simulink model "sampleModel258"  (R2021b)
settings: Solver=VariableStepAuto  StartTime=0.0  StopTime=10.0  RelTol=1e-3
undefined symbols (not defined in the file or in its folder): Newton, Raphson
libraries: simulink x13, slpidlib x2
settings Model: Creator=user  LastModifiedBy=user

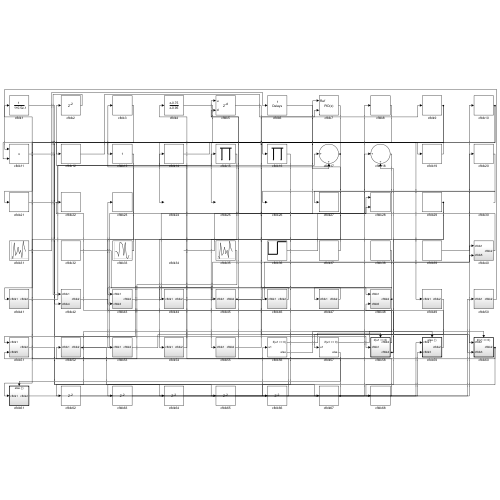
[thumbnail: Simulink's stored preview of the top-level diagram]
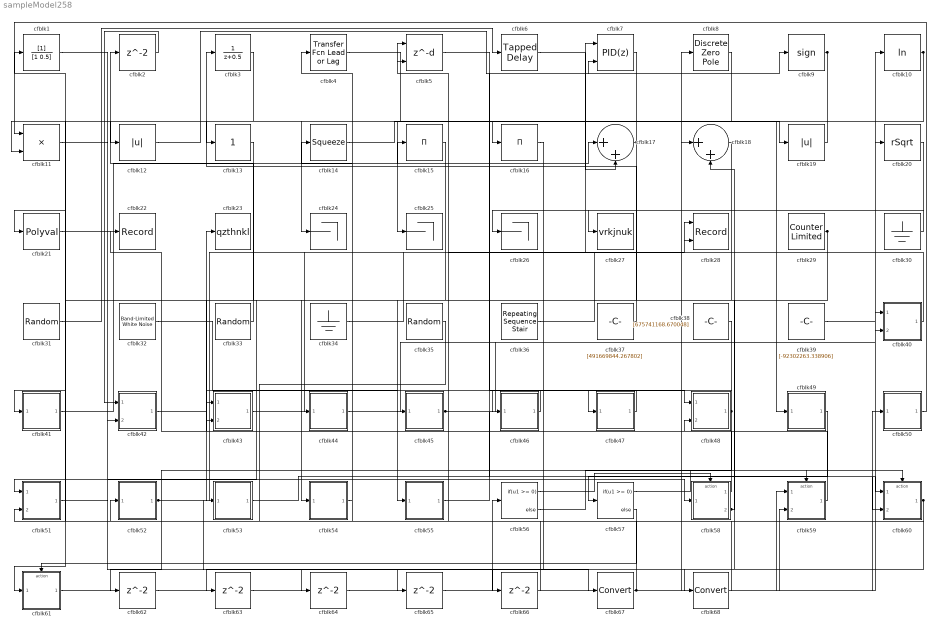
== system sampleModel258 ==
  cfblk1 : DiscreteFilter  SampleTime=1
  cfblk10 : Math  Operator=log  SaturateOnIntegerOverflow=on
  cfblk11 : Product  Inputs=**
  cfblk12 : Abs
  cfblk13 : simulink/Math Operations/Slider Gain  gain=1  low=0  high=2
  cfblk14 : Squeeze
  cfblk15 : Product  Inputs=*
  cfblk16 : Product  Inputs=*
  cfblk17 : Sum  Inputs=|++
  cfblk18 : Sum  Inputs=|++
  cfblk19 : Abs
  cfblk{2,62..66} (6 alike) : Delay  SampleTime=1
  cfblk20 : Sqrt  Operator=rSqrt  AlgorithmType=Newton-Raphson  SaturateOnIntegerOverflow=on
  cfblk21 : Polyval  Coefs=[ +2.081618890e-019, -1.441693666e-014, +4.719686976e-010, -8.536869453e-006, +1.621573104e-001, -8.087801117e+001 ]
  cfblk22 : Record  FileSettingsInternal="{\"entries\":[{\"content\":{\"excelSettings\":{\"content\":{},\"type\":\"Streamout.ExcelSettings\"}},\"type\":\"Streamout.FileSettingStorage\",\"uuid\":\"0ec8da23-2161-4a9d-a8a6-f1492471a594\"}],\"packageUris\":[\"http://schema.mathworks.com/mf0/streamout_blocks/R2020a\"],\"version\":\"1.0\"}"  SignalsInternal="{\"entries\":[{\"content\":{\"signals\":[{\"content\":{\"blockPath\":[\"sampleModel258/cfblk22\"],\"channel\":[],\"dimensions\":[1,1],\"domain\":\"sampleModel258/cfblk22\",\"lineColor\":\"#d95319\",\"plots\":[1],\"port\":1,\"sid\":[\"\"],\"signalID\":10667,\"signalName\":\"cfblk59\"},\"type\":\"RecordBlkView.Signal\",\"uuid\":\"13791875-5c6d-4bb0-95fb-77da70401f61\"}]},\"type\":\"RecordBlkView.InputSignals\",\"uuid\":\"91cc19b9-e580-4e4a-b56f-bdf48a70d35d\"}],\"packageUris\":[\"http://schema.mathworks.com/mf0/streamout_blocks/R2020a\"],\"version\":\"1.0\"}"  VisualizationBindings="{\"sparklinesplugin\":{\"info\":[{\"bindingParametersList\":[],\"subplotID\":1}]}}"
  cfblk23 : ToWorkspace  VariableName=qzthnkl  SaveFormat=Timeseries  SampleTime=-1
  cfblk24 : Terminator
  cfblk25 : Terminator
  cfblk26 : Terminator
  cfblk27 : ToWorkspace  VariableName=vrkjnuk  SaveFormat=Timeseries  SampleTime=-1
  cfblk28 : Record  FileSettingsInternal="{\"entries\":[{\"content\":{\"excelSettings\":{\"content\":{},\"type\":\"Streamout.ExcelSettings\"}},\"type\":\"Streamout.FileSettingStorage\",\"uuid\":\"56d646ea-4447-4100-bd41-ac8c1b7b2ac5\"}],\"packageUris\":[\"http://schema.mathworks.com/mf0/streamout_blocks/R2020a\"],\"version\":\"1.0\"}"  Layout=[1 1]  SignalsInternal="{\"entries\":[{\"content\":{\"signals\":[{\"content\":{\"blockPath\":[\"sampleModel258/cfblk28\"],\"channel\":[],\"dimensions\":[1],\"domain\":\"sampleModel258/cfblk28\",\"lineColor\":\"#a2142f\",\"plots\":[1],\"port\":1,\"sid\":[\"\"],\"signalID\":10671,\"signalName\":\"cfblk36\"},\"type\":\"RecordBlkView.Signal\",\"uuid\":\"d70a7a42-212c-47d6-9b85-39228d5a4333\"},{\"content\":{\"blockPath\":[\"sampleModel258/cfblk28\"],\"channel\":[],\"dimensions\":[1],\"domain\":\"sampleModel258/cfblk28\",\"lineColor\":\"#139fff\",\"plots\":[1],\"port\":2,\"sid\":[\"\"],\"signalID\":10675,\"signalName\":\"cfblk43\"},\"type\":\"RecordBlkView.Signal\",\"uuid\":\"f3014852-2a86-4845-a5c4-efbef73839ba\"}]},\"type\":\"RecordBlkView.InputSignals\",\"uuid\":\"fac5a7e7-c933-4a0b-812e-c4fec9d164f8\"}],\"packageUris\":[\"http://schema.mathworks.com/mf0/streamout_blocks/R2020a\"],\"version\":\"1.0\"}"  VisualizationBindings="{\"xyplotplugin\":{\"info\":[{\"series\":[{\"bindingParametersList\":[{\"parameter\":\"X-Axis\",\"signalID\":10671,\"signalName\":\"cfblk36\"},{\"parameter\":\"Y-Axis\",\"signalID\":10675,\"signalName\":\"cfblk43\"}],\"seriesID\":24969}],\"subplotID\":1}]}}"  CompatibilityTag=XY
  cfblk29 : simulink/Sources/Counter Limited  uplimit=[963.000000]  tsamp=-1
  cfblk3 : DiscreteTransferFcn  SampleTime=1
  cfblk30 : Ground
  cfblk31 : UniformRandomNumber  Minimum=[-523047582.222967]  Maximum=[2283029263.965306]  Seed=[18053115.000000]  SampleTime=0.1
  cfblk32 : simulink/Sources/Band-Limited White Noise  Cov=[465247779.470941]  Ts=0.1  seed=[5161787319.000000]
  cfblk33 : RandomNumber  Mean=[-77347.122146]  Variance=[42546.750938]  Seed=[226363169.000000]  SampleTime=0.1
  cfblk34 : Ground
  cfblk35 : UniformRandomNumber  Minimum=[-1875152426.312598]  Maximum=[3895215180.124573]  Seed=[16865050.000000]  SampleTime=0.1
  cfblk36 : simulink/Sources/Repeating Sequence Stair  OutValues=[-492891194.523507, -158957976.510578]  tsamp=-1  OutMin=[]  OutMax=[]  OutDataTypeStr=double  OutputDataTypeScalingMode=double  OutDataType=fixdt(0,8)  ConRadixGroup=Best Precision: Vector-wise  OutScaling=2^-12
  cfblk37 : Constant  Value=[491669844.267802]  SampleTime=1
  cfblk38 : Constant  Value=[675741168.670048]  SampleTime=1
  cfblk39 : Constant  Value=[-92302263.338906]  SampleTime=1
  cfblk4 : simulink/Discrete/Transfer Fcn Lead or Lag  PoleZ=0.95  ZeroZ=0.75  ICPrevOutput=0.0  ICPrevInput=0.0  DoSatur=off
      settings: SourceProductBaseCode=SL
  cfblk40 : Subsystem
  cfblk41 : Subsystem
  cfblk42 : Subsystem
  cfblk43 : Subsystem
  cfblk44 : Subsystem
  cfblk45 : Subsystem
  cfblk46 : Subsystem
  cfblk47 : Subsystem
  cfblk48 : Subsystem
  cfblk49 : Subsystem
  cfblk5 : Delay  DelayLengthSource=Input port  SampleTime=1
      settings: InputPortMap=u0,p1
  cfblk50 : Subsystem
  cfblk51 : Subsystem
  cfblk52 : Subsystem
  cfblk53 : Subsystem
  cfblk54 : Subsystem
  cfblk55 : Subsystem
  cfblk56 : If  IfExpression=u1 >= 0  SampleTime=1
  cfblk57 : If  IfExpression=u1 >= 0  SampleTime=1
  cfblk58 : Subsystem  TreatAsAtomicUnit=on
  cfblk59 : Subsystem  TreatAsAtomicUnit=on
  cfblk6 : simulink/Discrete/Tapped Delay  vinit=0.0  samptime=-1  NumDelays=1  DelayOrder=Oldest  includeCurrent=off
  cfblk60 : Subsystem  TreatAsAtomicUnit=on
  cfblk61 : Subsystem  TreatAsAtomicUnit=on
  cfblk67 : DataTypeConversion
  cfblk68 : DataTypeConversion
  cfblk7 : slpidlib/PID Controller (2DOF)  Controller=PID  Form=Parallel  TimeDomain=Discrete-time  UseExternalTs=off  SampleTime=1  IntegratorMethod=Forward Euler  FilterMethod=Forward Euler  ControllerParametersSource=internal  P=1  I=1  D=0  UseFilter=on  N=100  b=1  c=1  TunerSelectOption=Transfer Function Based (PID Tuner App)  InitialConditionSource=internal  InitialConditionForIntegrator=0  InitialConditionForFilter=0  DifferentiatorICPrevScaledInput=0  ExternalReset=none  TrackingMode=off  Kt=1  LimitOutput=off  SatLimitsSource=internal  UpperSaturationLimit=inf  LowerSaturationLimit=-inf  LinearizeAsGain=off  AntiWindupMode=none  Kb=1  POutMin=[]  POutMax=[]  IOutMin=[]  IOutMax=[]  DOutMin=[]  DOutMax=[]  NOutMin=[]  NOutMax=[]  bOutMin=[]  bOutMax=[]  cOutMin=[]  cOutMax=[]  SumOutMin=[]  SumOutMax=[]  SaturationOutMin=[]  SaturationOutMax=[]  PParamMin=[]  PParamMax=[]  IParamMin=[]  IParamMax=[]  DParamMin=[]  DParamMax=[]  NParamMin=[]  NParamMax=[]  bParamMin=[]  bParamMax=[]  cParamMin=[]  cParamMax=[]  KbParamMin=[]  KbParamMax=[]  KtParamMin=[]  KtParamMax=[]  KbOutMin=[]  KbOutMax=[]  KtOutMin=[]  KtOutMax=[]  IntegratorOutMin=[]  IntegratorOutMax=[]  FilterOutMin=[]  FilterOutMax=[]  SumI1OutMin=[]  SumI1OutMax=[]  SumI2OutMin=[]  SumI2OutMax=[]  SumI3OutMin=[]  SumI3OutMax=[]  SumI4OutMin=[]  SumI4OutMax=[]  SumDOutMin=[]  SumDOutMax=[]  Sum1OutMin=[]  Sum1OutMax=[]  Sum2OutMin=[]  Sum2OutMax=[]  Sum3OutMin=[]  Sum3OutMax=[]  DifferentiatorOutMin=[]  DifferentiatorOutMax=[]  FilterDiffOutCoefMin=[]  FilterDiffOutCoefMax=[]  ReciprocalOutMin=[]  ReciprocalOutMax=[]  SumDenOutMin=[]  SumDenOutMax=[]  SumNumOutMin=[]  SumNumOutMax=[]  DivideOutMin=[]  DivideOutMax=[]  UdiffTsProdOutMin=[]  UdiffTsProdOutMax=[]  NTsProdOutMin=[]  NTsProdOutMax=[]  UintegralTsProdOutMin=[]  UintegralTsProdOutMax=[]  UngainTsProdOutMin=[]  UngainTsProdOutMax=[]  IntegratorContinuousStateAttributes=''  IntegratorStateMustResolveToSignalObject=off  IntegratorRTWStateStorageClass=Auto  FilterContinuousStateAttributes=''  FilterStateMustResolveToSignalObject=off  FilterRTWStateStorageClass=Auto  ParallelPVariant=InternalParameters  IdealPVariant=Disabled  IVariant=InternalParameters  DVariant=InternalParameters  bVariant=InternalParameters  cVariant=InternalParameters  IntegratorVariant=Discrete  SatVariant=Disabled  AWVariant=Passthrough  PCopyVariant=Disabled  TRVariant=Disabled  FdbkBlocksVariant=Forward  IdealPFdbkVariant=Disabled  SatFdbkVariant=Disabled  DerivativeFilterVariant=ForwardEulerFilter  NVariant=InternalParameters  NCopyVariant=Disabled  FilterICVariant=InternalICsFilter  IntegratorICVariant=InternalICs  ExternalResetVariant=Disabled  TRSumVariant=Passthrough  SumFdbkVariant=Disabled  SumVariant=Sum_PID  TsampFilterVariant=InternalTs  TsampNgainVariant=Passthrough  TsampIntegralVariant=Passthrough  ExternalSaturationOutDataTypeStr=Inherit: Same as second input
      settings: SourceProductBaseCode=SL
  cfblk8 : DiscreteZeroPole  Poles=[0 0.5]  Gain=1
  cfblk9 : Signum
  wires:
  cfblk30/1 -> cfblk27/1
  cfblk10/1 -> cfblk25/1, cfblk11/2
  cfblk33/1 -> cfblk2/1
  cfblk39/1 -> cfblk10/1
  cfblk15/1 -> cfblk51/1(cfblk1)
  cfblk38/1 -> cfblk54/1(cfblk1)
  cfblk41/1(cfblk2) -> cfblk15/1
  cfblk2/1 -> cfblk42/1(cfblk1)
  cfblk9/1 -> cfblk24/1, cfblk42/2(cfblk4)
  cfblk60/1(cfblk2) -> cfblk52/1(cfblk1), cfblk63/1
  cfblk31/1 -> cfblk6/1
  cfblk36/1 -> cfblk28/1
  cfblk20/1 -> cfblk26/1
  cfblk61/1(cfblk2) -> cfblk20/1
  cfblk37/1 -> cfblk3/1
  cfblk48/1(cfblk2) -> cfblk47/1(cfblk1), cfblk62/1
  cfblk12/1 -> cfblk9/1
  cfblk50/1(cfblk2) -> cfblk11/1
  cfblk19/1 -> cfblk16/1
  cfblk7/1 -> cfblk12/1
  cfblk35/1 -> cfblk51/2(cfblk5)
  cfblk21/1 -> cfblk17/1
  cfblk6/1 -> cfblk17/2
  cfblk40/1(cfblk2) -> cfblk5/1
  cfblk14/1 -> cfblk19/1
  cfblk58/1(cfblk2) -> cfblk23/1
  cfblk8/1 -> cfblk41/1(cfblk1)
  cfblk1/1 -> cfblk67/1
  cfblk54/1(cfblk2) -> cfblk4/1
  cfblk17/1 -> cfblk13/1, cfblk45/1(cfblk1)
  cfblk52/1(cfblk2) -> cfblk8/1, cfblk65/1
  cfblk13/1 -> cfblk61/1(cfblk1)
  cfblk11/1 -> cfblk58/1(cfblk1)
  cfblk18/1 -> cfblk53/1(cfblk1)
  cfblk5/1 -> cfblk48/1(cfblk1)
  cfblk45/1(cfblk2) -> cfblk40/1(cfblk1), cfblk60/2(cfblk3)
  cfblk46/1(cfblk2) -> cfblk43/1(cfblk1)
  cfblk58/2(cfblk4) -> cfblk48/2(cfblk5), cfblk18/2
  cfblk43/1(cfblk2) -> cfblk28/2
  cfblk32/1 -> cfblk55/1(cfblk1)
  cfblk29/1 -> cfblk44/1(cfblk1), cfblk68/1
  cfblk4/1 -> cfblk49/1(cfblk1)
  cfblk34/1 -> cfblk7/1
  cfblk53/1(cfblk2) -> cfblk60/1(cfblk1)
  cfblk42/1(cfblk2) -> cfblk43/2(cfblk3)
  cfblk55/1(cfblk2) -> cfblk7/2
  cfblk47/1(cfblk2) -> cfblk46/1(cfblk1)
  cfblk49/1(cfblk2) -> cfblk57/1
  cfblk44/1(cfblk2) -> cfblk40/2(cfblk5)
  cfblk3/1 -> cfblk21/1
  cfblk59/1(cfblk2) -> cfblk22/1
  cfblk56/1 -> cfblk58/Action
  cfblk56/2 -> cfblk59/Action
  cfblk57/1 -> cfblk60/Action
  cfblk57/2 -> cfblk61/Action
  cfblk62/1 -> cfblk59/1(cfblk1)
  cfblk63/1 -> cfblk56/1
  cfblk51/1(cfblk2) -> cfblk64/1
  cfblk64/1 -> cfblk59/2(cfblk3)
  cfblk65/1 -> cfblk18/1
  cfblk16/1 -> cfblk66/1
  cfblk66/1 -> cfblk14/1
  cfblk67/1 -> cfblk5/2, cfblk50/1(cfblk1)
  cfblk68/1 -> cfblk1/1

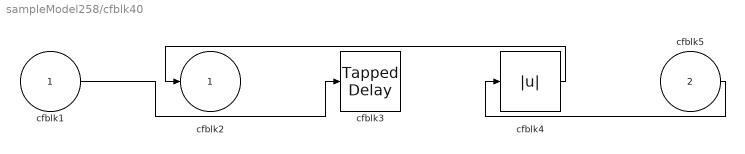
== system sampleModel258/cfblk40 ==
  cfblk1 : Inport
  cfblk5 : Inport  Port=2
  cfblk3 : simulink/Discrete/Tapped Delay  vinit=0.0  samptime=-1  NumDelays=1  DelayOrder=Oldest  includeCurrent=off
  cfblk4 : Abs
  cfblk2 : Outport
  wires:
  cfblk4/1 -> cfblk2/1
  cfblk1/1 -> cfblk3/1
  cfblk5/1 -> cfblk4/1

== system sampleModel258/cfblk41 ==
  cfblk1 : Inport
  cfblk3 : Abs
  cfblk2 : Outport
  wires:
  cfblk1/1 -> cfblk3/1
  cfblk3/1 -> cfblk2/1

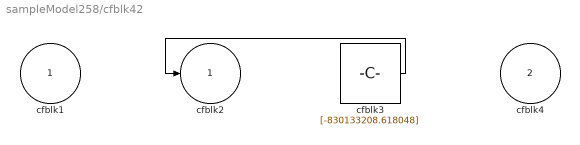
== system sampleModel258/cfblk42 ==
  cfblk1 : Inport
  cfblk4 : Inport  Port=2
  cfblk3 : Constant  Value=[-830133208.618048]  SampleTime=1
  cfblk2 : Outport
  wires:
  cfblk3/1 -> cfblk2/1

== system sampleModel258/cfblk43 ==
  cfblk1 : Inport
  cfblk3 : Inport  Port=2
  cfblk2 : Outport
  wires:
  cfblk3/1 -> cfblk2/1

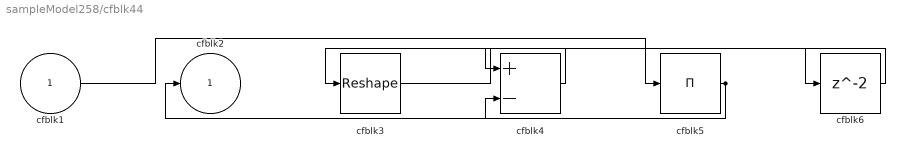
== system sampleModel258/cfblk44 ==
  cfblk1 : Inport
  cfblk3 : Reshape
  cfblk4 : Sum  Inputs=+-
  cfblk5 : Product  Inputs=*
  cfblk6 : Delay  SampleTime=1
  cfblk2 : Outport
  wires:
  cfblk4/1 -> cfblk3/1
  cfblk5/1 -> cfblk2/1, cfblk4/2
  cfblk1/1 -> cfblk5/1
  cfblk3/1 -> cfblk6/1
  cfblk6/1 -> cfblk4/1

== system sampleModel258/cfblk45 ==
  cfblk1 : Inport
  cfblk3 : Sum  Inputs=+-
  cfblk2 : Outport
  wires:
  cfblk1/1 -> cfblk3/1, cfblk3/2
  cfblk3/1 -> cfblk2/1

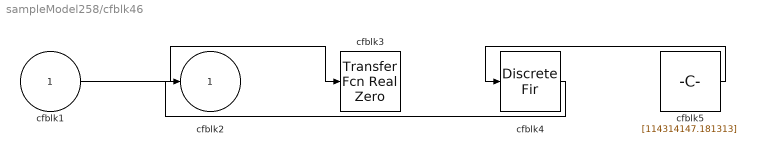
== system sampleModel258/cfblk46 ==
  cfblk1 : Inport
  cfblk3 : simulink/Discrete/Transfer Fcn Real Zero  ZeroZ=0.75  ICPrevInput=0.0  DoSatur=off
      settings: SourceProductBaseCode=SL
  cfblk4 : DiscreteFir  SampleTime=1
  cfblk5 : Constant  Value=[114314147.181313]  SampleTime=1
  cfblk2 : Outport
  wires:
  cfblk1/1 -> cfblk3/1
  cfblk5/1 -> cfblk4/1
  cfblk4/1 -> cfblk2/1

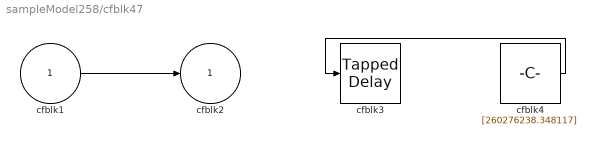
== system sampleModel258/cfblk47 ==
  cfblk1 : Inport
  cfblk3 : simulink/Discrete/Tapped Delay  vinit=0.0  samptime=-1  NumDelays=1  DelayOrder=Oldest  includeCurrent=off
  cfblk4 : Constant  Value=[260276238.348117]  SampleTime=1
  cfblk2 : Outport
  wires:
  cfblk4/1 -> cfblk3/1
  cfblk1/1 -> cfblk2/1

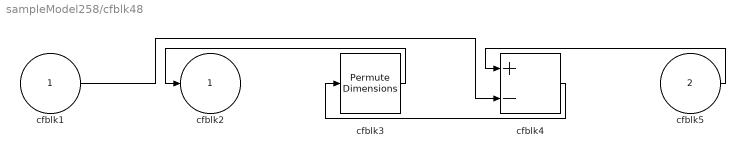
== system sampleModel258/cfblk48 ==
  cfblk1 : Inport
  cfblk5 : Inport  Port=2
  cfblk3 : PermuteDimensions
  cfblk4 : Sum  Inputs=+-
  cfblk2 : Outport
  wires:
  cfblk3/1 -> cfblk2/1
  cfblk4/1 -> cfblk3/1
  cfblk5/1 -> cfblk4/1
  cfblk1/1 -> cfblk4/2

== system sampleModel258/cfblk49 ==
  cfblk1 : Inport
  cfblk3 : simulink/Discrete/Tapped Delay  vinit=0.0  samptime=-1  NumDelays=1  DelayOrder=Oldest  includeCurrent=off
  cfblk2 : Outport
  wires:
  cfblk1/1 -> cfblk2/1, cfblk3/1

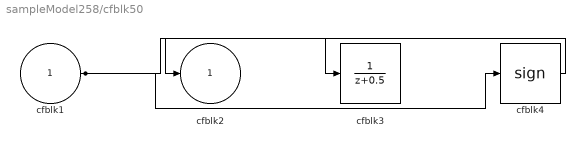
== system sampleModel258/cfblk50 ==
  cfblk1 : Inport
  cfblk3 : DiscreteTransferFcn  SampleTime=1
  cfblk4 : Signum
  cfblk2 : Outport
  wires:
  cfblk4/1 -> cfblk2/1
  cfblk1/1 -> cfblk4/1, cfblk3/1

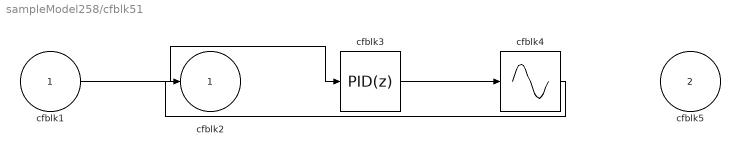
== system sampleModel258/cfblk51 ==
  cfblk1 : Inport
  cfblk5 : Inport  Port=2
  cfblk3 : slpidlib/PID Controller  Controller=PID  Form=Parallel  TimeDomain=Discrete-time  UseExternalTs=off  SampleTime=1  IntegratorMethod=Forward Euler  FilterMethod=Forward Euler  ControllerParametersSource=internal  P=1  I=1  D=0  UseFilter=on  N=100  TunerSelectOption=Transfer Function Based (PID Tuner App)  InitialConditionSource=internal  InitialConditionForIntegrator=0  InitialConditionForFilter=0  DifferentiatorICPrevScaledInput=0  ExternalReset=none  TrackingMode=off  Kt=1  LimitOutput=off  SatLimitsSource=internal  UpperSaturationLimit=inf  LowerSaturationLimit=-inf  LinearizeAsGain=off  AntiWindupMode=none  Kb=1  POutMin=[]  POutMax=[]  IOutMin=[]  IOutMax=[]  DOutMin=[]  DOutMax=[]  NOutMin=[]  NOutMax=[]  SumOutMin=[]  SumOutMax=[]  SaturationOutMin=[]  SaturationOutMax=[]  PParamMin=[]  PParamMax=[]  IParamMin=[]  IParamMax=[]  DParamMin=[]  DParamMax=[]  NParamMin=[]  NParamMax=[]  KbParamMin=[]  KbParamMax=[]  KtParamMin=[]  KtParamMax=[]  KbOutMin=[]  KbOutMax=[]  KtOutMin=[]  KtOutMax=[]  IntegratorOutMin=[]  IntegratorOutMax=[]  FilterOutMin=[]  FilterOutMax=[]  SumI1OutMin=[]  SumI1OutMax=[]  SumI2OutMin=[]  SumI2OutMax=[]  SumI3OutMin=[]  SumI3OutMax=[]  SumI4OutMin=[]  SumI4OutMax=[]  SumDOutMin=[]  SumDOutMax=[]  DifferentiatorOutMin=[]  DifferentiatorOutMax=[]  FilterDiffOutCoefMin=[]  FilterDiffOutCoefMax=[]  ReciprocalOutMin=[]  ReciprocalOutMax=[]  SumDenOutMin=[]  SumDenOutMax=[]  SumNumOutMin=[]  SumNumOutMax=[]  DivideOutMin=[]  DivideOutMax=[]  UdiffTsProdOutMin=[]  UdiffTsProdOutMax=[]  NTsProdOutMin=[]  NTsProdOutMax=[]  UintegralTsProdOutMin=[]  UintegralTsProdOutMax=[]  UngainTsProdOutMin=[]  UngainTsProdOutMax=[]  IntegratorContinuousStateAttributes=''  IntegratorStateMustResolveToSignalObject=off  IntegratorRTWStateStorageClass=Auto  FilterContinuousStateAttributes=''  FilterStateMustResolveToSignalObject=off  FilterRTWStateStorageClass=Auto  ParallelPVariant=InternalParameters  IdealPVariant=Disabled  IVariant=InternalParameters  DVariant=InternalParameters  IntegratorVariant=Discrete  SatVariant=Disabled  AWVariant=Passthrough  PCopyVariant=Disabled  TRVariant=Disabled  FdbkBlocksVariant=Forward  IdealPFdbkVariant=Disabled  SatFdbkVariant=Disabled  DerivativeFilterVariant=ForwardEulerFilter  NVariant=InternalParameters  NCopyVariant=Disabled  FilterICVariant=InternalICsFilter  IntegratorICVariant=InternalICs  ExternalResetVariant=Disabled  TRSumVariant=Passthrough  SumFdbkVariant=Disabled  SumVariant=Sum_PID  TsampFilterVariant=InternalTs  TsampNgainVariant=Passthrough  TsampIntegralVariant=Passthrough  ExternalSaturationOutDataTypeStr=Inherit: Same as second input
  cfblk4 : Sin  TimeSource=Use external signal  SampleTime=0
  cfblk2 : Outport
  wires:
  cfblk1/1 -> cfblk3/1
  cfblk3/1 -> cfblk4/1
  cfblk4/1 -> cfblk2/1

== system sampleModel258/cfblk52 ==
  cfblk1 : Inport
  cfblk3 : Constant  Value=[-294072416.670061]  SampleTime=1
  cfblk2 : Outport
  wires:
  cfblk1/1 -> cfblk2/1

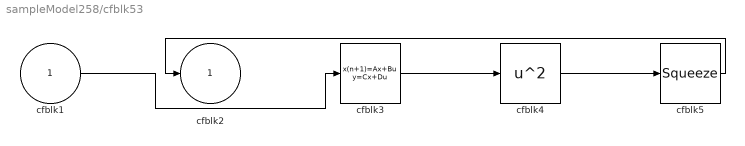
== system sampleModel258/cfblk53 ==
  cfblk1 : Inport
  cfblk3 : DiscreteStateSpace
  cfblk4 : Math  Operator=square  SaturateOnIntegerOverflow=on
  cfblk5 : Squeeze
  cfblk2 : Outport
  wires:
  cfblk5/1 -> cfblk2/1
  cfblk1/1 -> cfblk3/1
  cfblk3/1 -> cfblk4/1
  cfblk4/1 -> cfblk5/1

== system sampleModel258/cfblk54 ==
  cfblk1 : Inport
  cfblk3 : simulink/Discrete/Difference  ICPrevInput=0.0  OutMin=[]  OutMax=[]  OutDataTypeStr=Inherit: Inherit via back propagation  OutDataType=fixdt(1, 16)  OutScaling=2^-10  DoSatur=off
  cfblk4 : simulink/Discrete/Transfer Fcn Lead or Lag  PoleZ=0.95  ZeroZ=0.75  ICPrevOutput=0.0  ICPrevInput=0.0  DoSatur=off
      settings: SourceProductBaseCode=SL
  cfblk2 : Outport
  wires:
  cfblk3/1 -> cfblk2/1
  cfblk4/1 -> cfblk3/1
  cfblk1/1 -> cfblk4/1

== system sampleModel258/cfblk55 ==
  cfblk1 : Inport
  cfblk3 : Abs
  cfblk2 : Outport
  wires:
  cfblk1/1 -> cfblk2/1, cfblk3/1

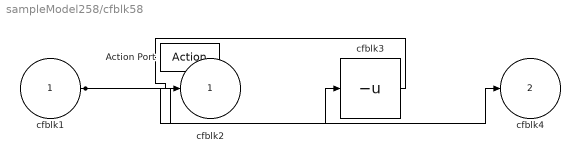
== system sampleModel258/cfblk58 ==
  cfblk1 : Inport
  Action Port : ActionPort  ActionPortLabel=if(u1 >= 0)
  cfblk3 : UnaryMinus
  cfblk2 : Outport
  cfblk4 : Outport  Port=2
  wires:
  cfblk1/1 -> cfblk4/1, cfblk3/1
  cfblk3/1 -> cfblk2/1

== system sampleModel258/cfblk59 ==
  cfblk1 : Inport
  cfblk3 : Inport  Port=2
  Action Port : ActionPort  ActionPortLabel=else
  cfblk2 : Outport
  wires:
  cfblk1/1 -> cfblk2/1

== system sampleModel258/cfblk60 ==
  cfblk1 : Inport
  cfblk3 : Inport  Port=2
  Action Port : ActionPort  ActionPortLabel=if(u1 >= 0)
  cfblk2 : Outport
  wires:
  cfblk3/1 -> cfblk2/1

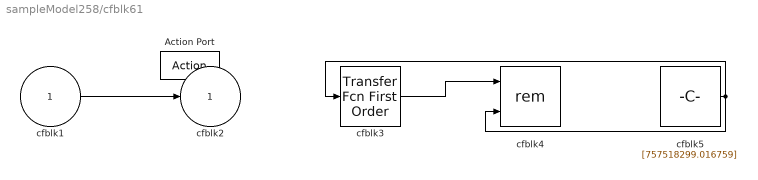
== system sampleModel258/cfblk61 ==
  cfblk1 : Inport
  Action Port : ActionPort  ActionPortLabel=else
  cfblk3 : simulink/Discrete/Transfer Fcn First Order  PoleZ=0.95  ICPrevOutput=0.0  DoSatur=off
  cfblk4 : Math  Operator=rem  SaturateOnIntegerOverflow=on
  cfblk5 : Constant  Value=[757518299.016759]  SampleTime=1
  cfblk2 : Outport
  wires:
  cfblk1/1 -> cfblk2/1
  cfblk5/1 -> cfblk3/1, cfblk4/2
  cfblk3/1 -> cfblk4/1
